simulink model "L0701"  (R2022b)
settings: Solver=FixedStepDiscrete  StartTime=0.0  StopTime=10.0  FixedStep=1  RelTol=1e-3
InitFcn:
  | inpdata
StopFcn:
  | outdialogs
settings Model: Creator=Andrey  LastModifiedBy=Andrey
settings DataIOCC: LimitDataPoints=on  MaxDataPoints=1  LoadExternalInput=on  SaveFormat=Array  SignalLogging=off  DSMLogging=off  SaveTime=off  ReturnWorkspaceOutputs=off

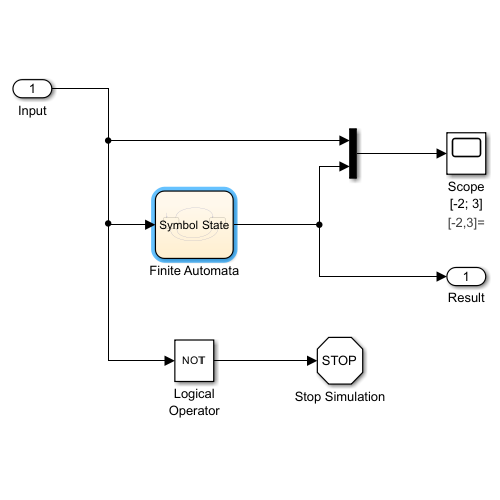
[thumbnail: Simulink's stored preview of the top-level diagram]
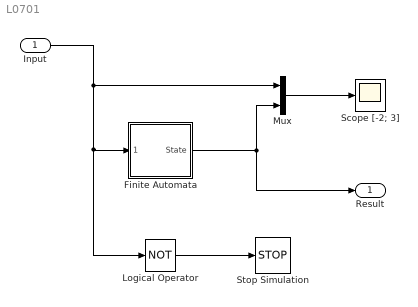
== system L0701 ==
  Input : Inport  SampleTime=1
  Finite Automata : Stateflow chart  TreatAsAtomicUnit=on
  Logical Operator : Logic  Operator=NOT  AllPortsSameDT=off  OutDataTypeStr=boolean
  Mux : Mux  Inputs=2
  Scope [-2; 3] : Scope
      settings: AttributesFormatString=[-2,3]=%<YLabel>
  Stop Simulation : Stop
  Result : Outport
  wires:
  Logical Operator/1 -> Stop Simulation/1
  Input/1 -> Mux/1, Finite Automata/1(Symbol), Logical Operator/1
  Finite Automata/1(State) -> Result/1, Mux/2
  Mux/1 -> Scope [-2; 3]/1

== stateflow chart L0701/Finite Automata ==
  state Zero
    entry: State = 0;
  state First
    entry:State=-1;
  Zero -> First : [Symbol == 1]
  (default) -> Zero
  First -> Zero [order 1] : [Symbol == 2]
  First -> Zero [order 2] : [Symbol == 1]
  data: Symbol input; State output
